simulink model "ieee_14_bus_system"  (R2022a)
settings: Solver=FixedStepDiscrete  StartTime=0.0  StopTime=T_final  FixedStep=T_sample  RelTol=1e-3
values from neighbouring files (symbols this model uses):
  A_bar_d = readmatrix('A_bar_d.csv')    [Run_model_WDS.m]
  B_bar_d = readmatrix('B_bar_d.csv')    [Run_model_WDS.m]
  C_obsv_d = readmatrix('C_obsv_d.csv')    [Run_model_WDS.m]    (also in run_model.m = C_obsv; run_model_power_system.m = C_obsv)
  D_obsv_d = readmatrix('D_obsv_d.csv')    [Run_model_WDS.m]    (also in run_model.m = D_obsv; run_model_power_system.m = D_obsv)
  H0_perp_full = eye(size(H0_full,1)) - H0_full*H0_full_pinv    [Run_model_WDS.m]    (also in run_model_power_system.m)
  load_buses = [zeros(n_gen,1); ones(n_bus-n_gen,1)]    [run_model.m]    (also in run_model_power_system.m)
  Lu = F-A_bar_d.'*H0_full_pinv*H1_full    [Run_model_WDS.m]    (also in run_model_power_system.m)
  Ly = A_bar_d.'*H0_full_pinv    [Run_model_WDS.m]    (also in run_model_power_system.m)
  n_bus = size(bus,1)    [run_model.m]    (also in run_model_power_system.m)
  n_gen = size(gen,1)    [run_model.m]    (also in run_model_power_system.m)
  n_states = 2*n_gen    [run_model.m]    (also in run_model_power_system.m)
  U0 = zeros(n_int,T+1)    [Run_model_WDS.m]    (also in run_model.m = zeros(m,T); run_model_power_system.m)
  x0 = zeros(n_states,1)    [Run_model_WDS.m]    (also in run_model.m; run_model_power_system.m)
  Y0 = zeros(n_meas,T)    [Run_model_WDS.m]    (also in run_model.m = zeros(m,T); run_model_power_system.m)
undefined symbols (not defined in the file or in its folder): H1_full, sigbuilder_block, T_start_opt
libraries: simulink x3
settings Model: Creator=Abelb  LastModifiedBy=Abelb

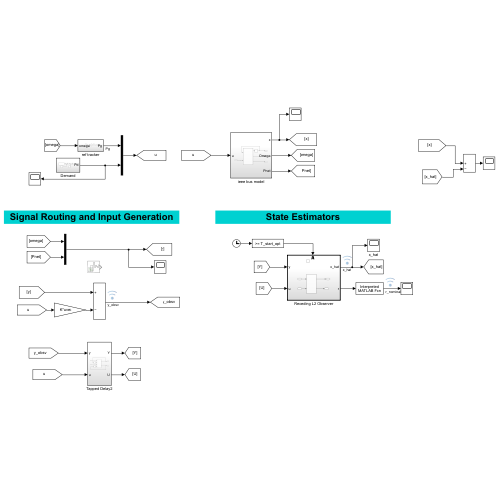
[thumbnail: Simulink's stored preview of the top-level diagram]
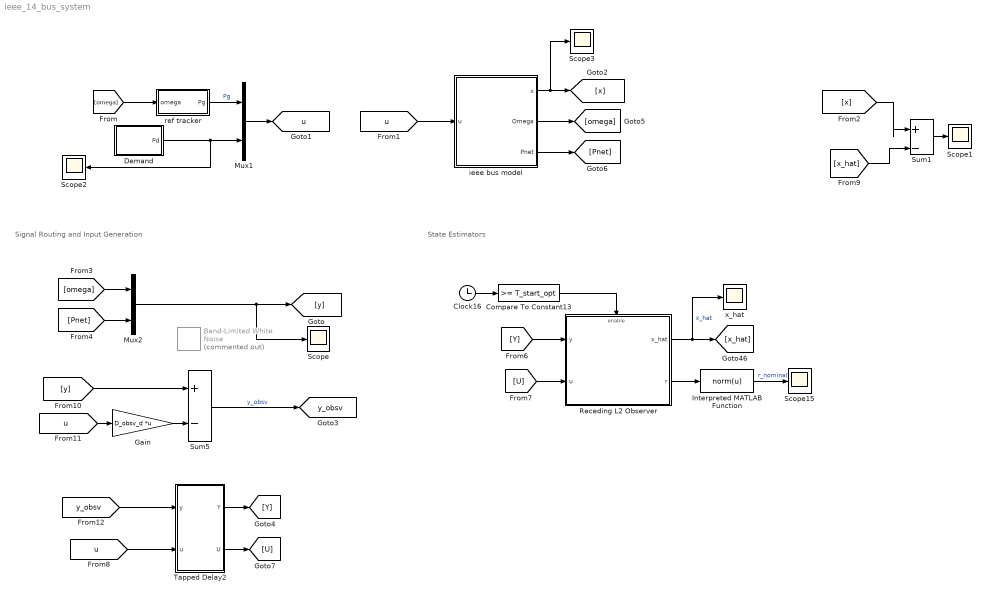
== system ieee_14_bus_system ==
  note: Signal Routing and Input Generation
  note: State Estimators
  Band-Limited White Noise : simulink/Sources/Band-Limited White Noise  Commented=on  Cov=1e-3  Ts=0.1  seed=[23341]
  Clock16 : Clock
  Compare To Constant13 : simulink/Logic and Bit Operations/Compare To Constant  relop=>=  const=T_start_opt  OutDataTypeStr=boolean
  Demand : Subsystem
  Gain : Gain  Gain=D_obsv_d  Multiplication=Matrix(K*u) (u vector)
  Interpreted MATLAB Function : MATLABFcn  MATLABFcn=norm(u)
  Mux1 : Mux  Inputs=2
  Mux2 : Mux  Inputs=2
  Receding L2 Observer : Subsystem
  Scope{,1..3,15} (5 alike) : Scope
  Sum1 : Sum  Inputs=|+-
  Sum5 : Sum  Inputs=+-
  Tapped Delay2 : Subsystem
  ieee bus model : Subsystem
  ref tracker : Subsystem
  x_hat : Scope
  tag scope: u=global, y_obsv=global
  wires:
  ref tracker/1(Pg) -> Mux1/1  "Pg"
  [u] -> ieee bus model/1(u)
  ieee bus model/2(Omega) -> [omega]
  ieee bus model/3(Pnet) -> [Pnet]
  Demand/1(Pd) -> Scope2/1, Mux1/2
  Mux1/1 -> [u]
  [omega] -> ref tracker/1(omega)
  ieee bus model/1(x) -> Scope3/1, [x]
  [Pnet] -> Mux2/2
  Mux2/1 -> Scope/1, [y]
  [omega] -> Mux2/1
  [y_obsv] -> Tapped Delay2/1(y)
  [u] -> Tapped Delay2/2(u)
  Tapped Delay2/2(U) -> [U]
  Tapped Delay2/1(Y) -> [Y]
  Receding L2 Observer/2(r) -> Interpreted MATLAB Function/1
  Interpreted MATLAB Function/1 -> Scope15/1  "r_nominal"
  [U] -> Receding L2 Observer/2(u)
  [Y] -> Receding L2 Observer/1(y)
  Clock16/1 -> Compare To Constant13/1
  Compare To Constant13/1 -> Receding L2 Observer/Enable
  Receding L2 Observer/1(x_hat) -> x_hat/1, [x_hat]  "x_hat"
  Sum1/1 -> Scope1/1
  [x_hat] -> Sum1/2
  [x] -> Sum1/1
  Sum5/1 -> [y_obsv]  "y_obsv"
  [u] -> Gain/1
  [y] -> Sum5/1
  Gain/1 -> Sum5/2

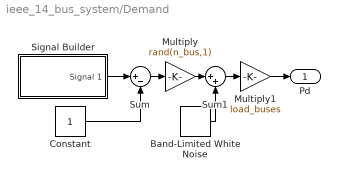
== system ieee_14_bus_system/Demand ==
  Band-Limited White Noise : simulink/Sources/Band-Limited White Noise  Cov=1e-8  Ts=0.1  seed=[23341]
  Constant : Constant
  Multiply : Gain  Gain=rand(n_bus,1)
  Multiply1 : Gain  Gain=load_buses
  Signal Builder : Subsystem  Tag=STV Subsys  LoadFcn=sigbuilder_block('load');  StartFcn=sigbuilder_block('start');  StopFcn=sigbuilder_block('stop');  ClipboardFcn=sigbuilder_block('clipboard');  mask(Sigbuilder block){tuvar=[0:10]}
      mask help: Simulink:masks:SigbuilderBlock_MD
      mask init:
      | if ~strcmp(get_param(bdroot(gcbh),'SimulationStatus'),'stopped') tuvar = sigbuilder_block('maskInit'); end
      settings: CopyFcn=sigbuilder_block('copy');  DeleteFcn=sigbuilder_block('delete');  ModelCloseFcn=sigbuilder_block('modelClose');  PreSaveFcn=sigbuilder_block('preSave');  PauseFcn=sigbuilder_block('pause');  ContinueFcn=sigbuilder_block('continue');  NameChangeFcn=sigbuilder_block('namechange');  OpenFcn=sigbuilder_block('open',[439.2 145.2 550.2 399.9 ]);  CloseFcn=sigbuilder_block('close');
      mask Display: plot(0, 0, 100, 100,[2, 2, 32, 32, 2], [68, 8, 8, 68, 68],[32, 2], [38, 38], [32, 19, 2],[53, 60, 44], [32, 17, 17, 2],[16, 16, 31, 31]);txt = getActiveGroup(gcbh);text(2, 100, txt,'verticalAlignment', 'top');
  Sum : Sum  Inputs=|+-
  Sum1 : Sum  Inputs=|++
  Pd : Outport
  wires:
  Sum/1 -> Multiply/1
  Signal Builder/1(Signal 1) -> Sum/1
  Constant/1 -> Sum/2
  Multiply/1 -> Sum1/1
  Band-Limited White Noise/1 -> Sum1/2
  Sum1/1 -> Multiply1/1
  Multiply1/1 -> Pd/1

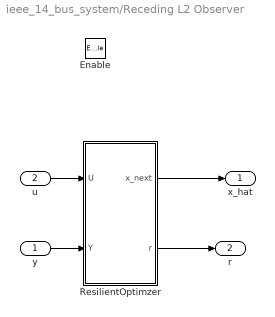
== system ieee_14_bus_system/Receding L2 Observer ==
  y : Inport
  u : Inport  Port=2
  Enable : EnablePort
  ResilientOptimzer : MATLAB Function  TreatAsAtomicUnit=on
  x_hat : Outport
  r : Outport  Port=2
  wires:
  y/1 -> ResilientOptimzer/2(Y)
  u/1 -> ResilientOptimzer/1(U)
  ResilientOptimzer/1(x_next) -> x_hat/1
  ResilientOptimzer/2(r) -> r/1

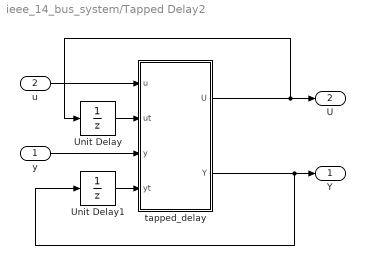
== system ieee_14_bus_system/Tapped Delay2 ==
  y : Inport
  u : Inport  Port=2
  Unit Delay : UnitDelay  InitialCondition=U0  SampleTime=-1  HasFrameUpgradeWarning=on
  Unit Delay1 : UnitDelay  InitialCondition=Y0  SampleTime=-1  HasFrameUpgradeWarning=on
  tapped_delay : MATLAB Function  TreatAsAtomicUnit=on
  Y : Outport
  U : Outport  Port=2
  wires:
  u/1 -> tapped_delay/1(u)
  y/1 -> tapped_delay/3(y)
  tapped_delay/1(U) -> Unit Delay/1, U/1
  tapped_delay/2(Y) -> Unit Delay1/1, Y/1
  Unit Delay/1 -> tapped_delay/2(ut)
  Unit Delay1/1 -> tapped_delay/4(yt)

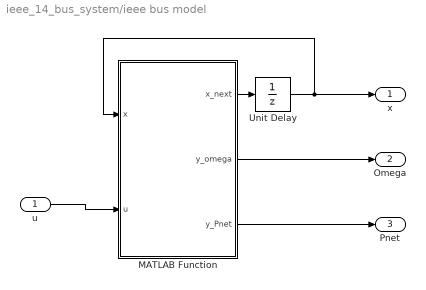
== system ieee_14_bus_system/ieee bus model ==
  u : Inport
  MATLAB Function : MATLAB Function  TreatAsAtomicUnit=on
  Unit Delay : UnitDelay  InitialCondition=x0  SampleTime=-1  HasFrameUpgradeWarning=on
  x : Outport
  Omega : Outport  Port=2
  Pnet : Outport  Port=3
  wires:
  MATLAB Function/1(x_next) -> Unit Delay/1
  Unit Delay/1 -> x/1, MATLAB Function/1(x)
  u/1 -> MATLAB Function/2(u)
  MATLAB Function/2(y_omega) -> Omega/1
  MATLAB Function/3(y_Pnet) -> Pnet/1

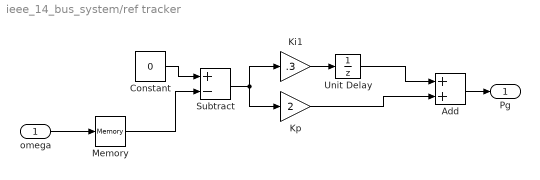
== system ieee_14_bus_system/ref tracker ==
  omega : Inport
  Add : Sum
  Constant : Constant  Value=0
  Ki1 : Gain  Gain=.3
  Kp : Gain  Gain=2
  Memory : Memory  InitialCondition=zeros(n_gen,1)
  Subtract : Sum  Inputs=+-
  Unit Delay : UnitDelay  InitialCondition=zeros(n_gen,1)  SampleTime=-1  HasFrameUpgradeWarning=on
  Pg : Outport
  wires:
  Kp/1 -> Add/2
  Unit Delay/1 -> Add/1
  Add/1 -> Pg/1
  Constant/1 -> Subtract/1
  Subtract/1 -> Ki1/1, Kp/1
  Ki1/1 -> Unit Delay/1
  Memory/1 -> Subtract/2
  omega/1 -> Memory/1

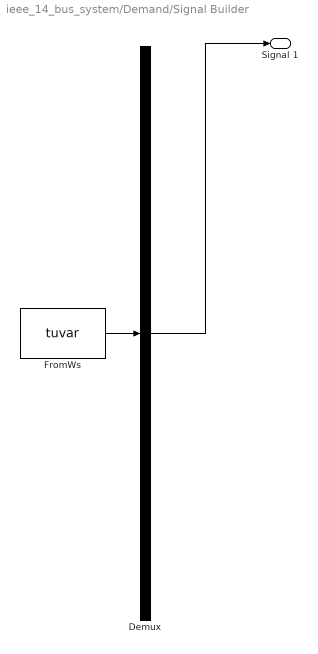
== system ieee_14_bus_system/Demand/Signal Builder ==
  Demux : Demux  Tag=STV Demux  Outputs=1
      settings: DisplayOption=none
  FromWs : FromWorkspace  Tag=STV FromWs  VariableName=tuvar
      SigBuilderData=|
      | common.afterFinalStr = 'Extrapolate'
      | common.sampleTime = 0
      | dataSet.timeRange = [0 10]
      | dataSet.name = 'Group 1'
      | sbobj.Groups.Name = 'Group 1'
      | sbobj.Groups.Signals.Name = 'Signal 1'
      | sbobj.Groups.Signals.XData = [0 0.46 1.5 2.5 4 5 6 7 10]
      | sbobj.Groups.Signals.YData = [1 1.106 1.2 1.2 0.8 0.8 1 1 1]
  Signal 1 : Outport  Tag=STV Outport
  wires:
  Demux/1 -> Signal 1/1
  FromWs/1 -> Demux/1

== matlab function ieee_14_bus_system/Tapped Delay2/tapped_delay ==
  data: u input; U output; ut input; y input; yt input; Y output
function [U,Y] = fcn(u,ut,y,yt)
%% tapped_delay_array
% shift columns from tapped matrix to the left and appends most recent
% vector to the last column
%%% input
ut(:,1:end-1) = ut(:,2:end);
ut(:,end) = u;
U = ut;
%%% output
yt(:,1:end-1) = yt(:,2:end);
yt(:,end) = y;
Y = yt;

== matlab function ieee_14_bus_system/ieee bus model/MATLAB Function ==
  data: x input; x_next output; u input; y_omega output; A_bar_d parameter; C_obsv_d parameter; B_bar_d parameter; D_obsv_d parameter; n_gen parameter; n_bus parameter; y_Pnet output
function [x_next,y_omega,y_Pnet] = fcn(x,u,A_bar_d,C_obsv_d,B_bar_d,D_obsv_d,n_gen, n_bus)
% Discrete state-space model for system

x_next = A_bar_d*x + B_bar_d*u;

y = C_obsv_d*x + D_obsv_d*u;

y_omega = y(1:n_gen);
y_Pnet = y(n_gen+1:n_bus+n_gen);

== matlab function ieee_14_bus_system/Receding L2 Observer/ResilientOptimzer ==
  data: x_next output; U input; Y input; Ly parameter; Lu parameter; H0_perp_full parameter; H1_full parameter; r output; n_states parameter
function [x_next,r]  = fcn(U,Y, Ly, Lu,H0_perp_full, H1_full,n_states)


u_local = U(:,1:end-1);
% vectorized
u = u_local(:);
y = Y(:);

x_next = zeros(n_states,1);
x_next(:) = Ly*y + Lu*u;

r = H0_perp_full*(y-H1_full*u);
